simulink model "MotorModel"  (R2019b)
settings: Solver=FixedStepAuto  StartTime=0.0  StopTime=50  FixedStep=0.01  RelTol=1e-3
undefined symbols (not defined in the file): IL, KB, KT, L, R
settings Model: Creator=Harun Berk Işık  LastModifiedBy=Harun Berk Işık

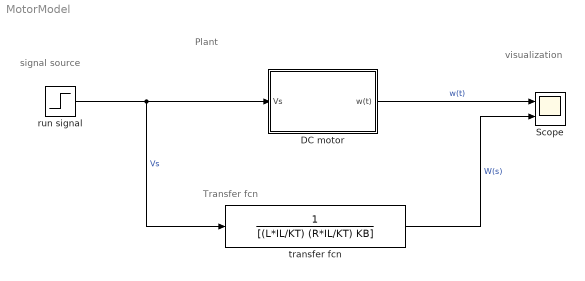
== system MotorModel ==
  note: visualization
  note: Transfer fcn
  note: signal source
  note: Plant
  DC motor : Subsystem
  Scope : Scope  NumInputPorts=2
  run signal : Step  Time=5  After=3  SampleTime=0
  "transfer fcn " : TransferFcn  Denominator=[(L*IL/KT) (R*IL/KT) KB]
  wires:
  run signal/1 -> "transfer fcn "/1, DC motor/1("Vs ")  "Vs"
  DC motor/1("w(t) ") -> Scope/1  "w(t)"
  "transfer fcn "/1 -> Scope/2  "W(s)"

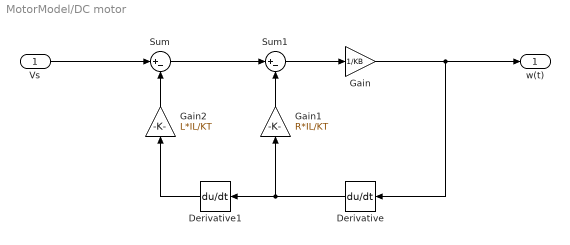
== system MotorModel/DC motor ==
  "Vs " : Inport
  Derivative : Derivative
  Derivative1 : Derivative
  Gain : Gain  Gain=1/KB
  Gain1 : Gain  Gain=R*IL/KT
  Gain2 : Gain  Gain=L*IL/KT
  Sum : Sum  Inputs=|+-
  Sum1 : Sum  Inputs=|+-
  "w(t) " : Outport
  wires:
  Gain/1 -> "w(t) "/1, Derivative/1
  Derivative/1 -> Gain1/1, Derivative1/1
  Sum1/1 -> Gain/1
  Sum/1 -> Sum1/1
  Gain1/1 -> Sum1/2
  Derivative1/1 -> Gain2/1
  Gain2/1 -> Sum/2
  "Vs "/1 -> Sum/1
